simulink model "Table_airbus_v1"  (R2021b)
settings: Solver=VariableStepAuto  StartTime=0.0  StopTime=20  MaxStep=0.01  RelTol=0.01
undefined symbols (not defined in the file): X, Y, Z
libraries: sm_lib x907, fl_lib x69, nesl_utility x53, sdl_lib x10, ee_lib x7, slpidlib x6, simulink x5, simulink_extras x4
(part 16 of 18)

== system Table_airbus_v1/Modèle mécanique/Table/table_1_RIGID/x15060_M_01014_Ens_plateau_Default_1_RIGID/x15060_M_01003_Ens_structure_plateau_Default_1_RIGID ==
  ReferenceFrame : sm_lib/Frames and Transforms/Reference Frame
  Transform : sm_lib/Frames and Transforms/Rigid Transform  TranslationMethod=Cartesian  TranslationStandardOffset=0  TranslationLengthUnit=mm  TranslationStandardAxis=+Z  TranslationCartesianOffset=[860 265 20]  TranslationROffset=0  TranslationROffsetUnits=m  TranslationZOffset=0  TranslationZOffsetUnits=m  TranslationThetaOffset=0  TranslationThetaOffsetUnits=deg  RotationMethod=ArbitraryAxis  RotationAngleUnits=rad  RotationStandardAxis=+Z  RotationAngle=2.0943951023931953  RotationArbitraryAxis=[-0.57735026918962584 0.57735026918962584 0.57735026918962584]  FollAlignAxisA=+X  BaseAlignAxisA=+Y  FollAlignAxisB=+Y  BaseAlignAxisB=+Z  RotationSequenceAxes=FollowerAxes  RotationSequence=XYX  RotationSequenceAngles=[0 0 0]  RotationSequenceAnglesUnits=deg  RotationMatrix=[1 0 0; 0 1 0; 0 0 1]
  Transform1 : sm_lib/Frames and Transforms/Rigid Transform  TranslationMethod=Cartesian  TranslationStandardOffset=0  TranslationLengthUnit=mm  TranslationStandardAxis=+Z  TranslationCartesianOffset=[860 -375 0]  TranslationROffset=0  TranslationROffsetUnits=m  TranslationZOffset=0  TranslationZOffsetUnits=m  TranslationThetaOffset=0  TranslationThetaOffsetUnits=deg  RotationMethod=ArbitraryAxis  RotationAngleUnits=rad  RotationStandardAxis=+Z  RotationAngle=1.5707963267948968  RotationArbitraryAxis=[-5.5510999999999988e-17 5.5510999999999988e-17 1]  FollAlignAxisA=+X  BaseAlignAxisA=+Y  FollAlignAxisB=+Y  BaseAlignAxisB=+Z  RotationSequenceAxes=FollowerAxes  RotationSequence=XYX  RotationSequenceAngles=[0 0 0]  RotationSequenceAnglesUnits=deg  RotationMatrix=[1 0 0; 0 1 0; 0 0 1]
  Transform2 : sm_lib/Frames and Transforms/Rigid Transform  TranslationMethod=None  TranslationStandardOffset=0  TranslationLengthUnit=m  TranslationStandardAxis=+Z  TranslationCartesianOffset=[0 0 0]  TranslationROffset=0  TranslationROffsetUnits=m  TranslationZOffset=0  TranslationZOffsetUnits=m  TranslationThetaOffset=0  TranslationThetaOffsetUnits=deg  RotationMethod=None  RotationAngleUnits=deg  RotationStandardAxis=+Z  RotationAngle=0  RotationArbitraryAxis=[0 0 1]  FollAlignAxisA=+X  BaseAlignAxisA=+Y  FollAlignAxisB=+Y  BaseAlignAxisB=+Z  RotationSequenceAxes=FollowerAxes  RotationSequence=XYX  RotationSequenceAngles=[0 0 0]  RotationSequenceAnglesUnits=deg  RotationMatrix=[1 0 0; 0 1 0; 0 0 1]
  Transform3 : sm_lib/Frames and Transforms/Rigid Transform  TranslationMethod=Cartesian  TranslationStandardOffset=0  TranslationLengthUnit=mm  TranslationStandardAxis=+Z  TranslationCartesianOffset=[860 375 5.5217500000000003e-09]  TranslationROffset=0  TranslationROffsetUnits=m  TranslationZOffset=0  TranslationZOffsetUnits=m  TranslationThetaOffset=0  TranslationThetaOffsetUnits=deg  RotationMethod=ArbitraryAxis  RotationAngleUnits=rad  RotationStandardAxis=+Z  RotationAngle=3.1415926535897931  RotationArbitraryAxis=[0.70710678118654768 -0.70710678118654735 0]  FollAlignAxisA=+X  BaseAlignAxisA=+Y  FollAlignAxisB=+Y  BaseAlignAxisB=+Z  RotationSequenceAxes=FollowerAxes  RotationSequence=XYX  RotationSequenceAngles=[0 0 0]  RotationSequenceAnglesUnits=deg  RotationMatrix=[1 0 0; 0 1 0; 0 0 1]
  Transform4 : sm_lib/Frames and Transforms/Rigid Transform  TranslationMethod=None  TranslationStandardOffset=0  TranslationLengthUnit=m  TranslationStandardAxis=+Z  TranslationCartesianOffset=[0 0 0]  TranslationROffset=0  TranslationROffsetUnits=m  TranslationZOffset=0  TranslationZOffsetUnits=m  TranslationThetaOffset=0  TranslationThetaOffsetUnits=deg  RotationMethod=ArbitraryAxis  RotationAngleUnits=rad  RotationStandardAxis=+Z  RotationAngle=3.1415926535897931  RotationArbitraryAxis=[-6.3838000000000003e-16 1.3216950000000001e-15 -1]  FollAlignAxisA=+X  BaseAlignAxisA=+Y  FollAlignAxisB=+Y  BaseAlignAxisB=+Z  RotationSequenceAxes=FollowerAxes  RotationSequence=XYX  RotationSequenceAngles=[0 0 0]  RotationSequenceAnglesUnits=deg  RotationMatrix=[1 0 0; 0 1 0; 0 0 1]
  x15060_ITEM_Kit_Equerre_8_40x40_Zn_0_0_411_15_AA_DEFAULT_1_RIGI : Subsystem
  x15060_ITEM_Kit_Equerre_8_80x80_Zn_0_0_411_32_AA_DEFAULT_1_RIGI : Subsystem
  x15060_ITEM_Kit_Equerre_8_80x80_Zn_0_0_411_32_AA_DEFAULT_2_RIGI : Subsystem
  x15060_M_01021_Plateau_en_profil_alu_40x40_AA_DEFAULT_Brut_dusi : Subsystem
  F : PMIOPort  Side=Right
  connections:
  Transform4/LConn1 -- F/RConn1
  Transform4/RConn1 -- Transform3/LConn1 -- Transform2/LConn1 -- Transform1/LConn1 -- ReferenceFrame/RConn1 -- Transform/LConn1
  Transform3/RConn1 -- x15060_ITEM_Kit_Equerre_8_80x80_Zn_0_0_411_32_AA_DEFAULT_2_RIGI/LConn1
  Transform2/RConn1 -- x15060_M_01021_Plateau_en_profil_alu_40x40_AA_DEFAULT_Brut_dusi/LConn1
  Transform1/RConn1 -- x15060_ITEM_Kit_Equerre_8_80x80_Zn_0_0_411_32_AA_DEFAULT_1_RIGI/LConn1
  Transform/RConn1 -- x15060_ITEM_Kit_Equerre_8_40x40_Zn_0_0_411_15_AA_DEFAULT_1_RIGI/LConn1

== system Table_airbus_v1/Modèle mécanique/Table/table_1_RIGID/x15060_M_01014_Ens_plateau_Default_1_RIGID/x15060_M_01022_Plaque_sup_plateau_AA_DEFAULT_1_RIGID ==
  ReferenceFrame : sm_lib/Frames and Transforms/Reference Frame
  Solid : sm_lib/Body Elements/File Solid  ExtGeomFileName=15060-M-01022-Plaque sup plateau_AA - DEFAULT_Défaut_sldprt.STL  UnitType=Custom  ExtGeomFileUnits=mm  StepReaderType=HEX  ExportConvexHullGeometry=off  InertiaType=Custom  Mass=17.528600000000001  MassUnits=kg  CenterOfMass=[0 0 10.5]  CenterOfMassUnits=mm  MomentsOfInertia=[1002910 4728250 5729860]  MomentsOfInertiaUnits=kg*mm^2  ProductsOfInertia=[0 0 0]  ProductsOfInertiaUnits=kg*mm^2  BasedOnType=Density  Density=1000  DensityUnits=kg/(m^3)  DoExposeReferenceFrame=on  SerializedFrames=<Frames/>  GraphicType=FromGeometry  MarkerShape=Sphere  MarkerSize=10  MarkerSizeUnits=m  GraphicVisPropType=SimpleVisualProperties  GraphicDiffuseColor=[1 1 1]  GraphicSpecularColor=[0.5 0.5 0.5 1.0]  GraphicAmbientColor=[0.15 0.15 0.15 1.0]  GraphicEmissiveColor=[0.0 0.0 0.0 1.0]  GraphicShininess=75  GraphicOpacity=1
  F : PMIOPort  Side=Left
  connections:
  F/RConn1 -- ReferenceFrame/RConn1 -- Solid/RConn1

== system Table_airbus_v1/Modèle mécanique/Table/table_1_RIGID/x15060_M_01014_Ens_plateau_Default_1_RIGID/x15060_M_01024_Cale_reglet_AA_DEFAULT_1_RIGID ==
  ReferenceFrame : sm_lib/Frames and Transforms/Reference Frame
  Solid : sm_lib/Body Elements/File Solid  ExtGeomFileName=15060-M-01024-Cale reglet_AA - DEFAULT_Défaut_sldprt.STL  UnitType=Custom  ExtGeomFileUnits=mm  StepReaderType=HEX  ExportConvexHullGeometry=off  InertiaType=Custom  Mass=0.00835726  MassUnits=kg  CenterOfMass=[0 0 5]  CenterOfMassUnits=mm  MomentsOfInertia=[0.72748299999999999 0.68167800000000001 1.2698699999999998]  MomentsOfInertiaUnits=kg*mm^2  ProductsOfInertia=[0 0 0]  ProductsOfInertiaUnits=kg*mm^2  BasedOnType=Density  Density=1000  DensityUnits=kg/(m^3)  DoExposeReferenceFrame=on  SerializedFrames=<Frames/>  GraphicType=FromGeometry  MarkerShape=Sphere  MarkerSize=10  MarkerSizeUnits=m  GraphicVisPropType=SimpleVisualProperties  GraphicDiffuseColor=[0.792157 0.819608 0.933333]  GraphicSpecularColor=[0.5 0.5 0.5 1.0]  GraphicAmbientColor=[0.15 0.15 0.15 1.0]  GraphicEmissiveColor=[0.0 0.0 0.0 1.0]  GraphicShininess=75  GraphicOpacity=1
  F : PMIOPort  Side=Left
  connections:
  F/RConn1 -- ReferenceFrame/RConn1 -- Solid/RConn1

== system Table_airbus_v1/Modèle mécanique/Table/table_1_RIGID/x15060_M_01014_Ens_plateau_Default_1_RIGID/x15060_M_01032_Porte_pivot_AA_DEFAULT_1_RIGID ==
  ReferenceFrame : sm_lib/Frames and Transforms/Reference Frame
  Solid : sm_lib/Body Elements/File Solid  ExtGeomFileName=15060-M-01032-Porte pivot_AA - DEFAULT_Défaut_sldprt.STL  UnitType=Custom  ExtGeomFileUnits=mm  StepReaderType=HEX  ExportConvexHullGeometry=off  InertiaType=Custom  Mass=0.45541399999999999  MassUnits=kg  CenterOfMass=[-47.106400000000001 48.122499999999995 0.36210500000000001]  CenterOfMassUnits=mm  MomentsOfInertia=[388.97500000000002 432.13300000000004 691.03600000000006]  MomentsOfInertiaUnits=kg*mm^2  ProductsOfInertia=[-6.7267999999999999 6.8385800000000003 -294.24299999999999]  ProductsOfInertiaUnits=kg*mm^2  BasedOnType=Density  Density=1000  DensityUnits=kg/(m^3)  DoExposeReferenceFrame=on  SerializedFrames=<Frames/>  GraphicType=FromGeometry  MarkerShape=Sphere  MarkerSize=10  MarkerSizeUnits=m  GraphicVisPropType=SimpleVisualProperties  GraphicDiffuseColor=[0.898039 0.917647 0.929412]  GraphicSpecularColor=[0.5 0.5 0.5 1.0]  GraphicAmbientColor=[0.15 0.15 0.15 1.0]  GraphicEmissiveColor=[0.0 0.0 0.0 1.0]  GraphicShininess=75  GraphicOpacity=1
  F : PMIOPort  Side=Left
  connections:
  F/RConn1 -- ReferenceFrame/RConn1 -- Solid/RConn1

== system Table_airbus_v1/Modèle mécanique/Table/table_1_RIGID/x15060_M_01014_Ens_plateau_Default_1_RIGID/x15060_M_01034_Axe_pivot_AA_DEFAULT_1_RIGID ==
  ReferenceFrame : sm_lib/Frames and Transforms/Reference Frame
  Solid : sm_lib/Body Elements/File Solid  ExtGeomFileName=15060-M-01034-Axe pivot_AA - DEFAULT_Défaut_sldprt.STL  UnitType=Custom  ExtGeomFileUnits=mm  StepReaderType=HEX  ExportConvexHullGeometry=off  InertiaType=Custom  Mass=0.12033099999999999  MassUnits=kg  CenterOfMass=[0 0 0]  CenterOfMassUnits=mm  MomentsOfInertia=[3.38402 4651.21 4651.21]  MomentsOfInertiaUnits=kg*mm^2  ProductsOfInertia=[0 0 0]  ProductsOfInertiaUnits=kg*mm^2  BasedOnType=Density  Density=1000  DensityUnits=kg/(m^3)  DoExposeReferenceFrame=on  SerializedFrames=<Frames/>  GraphicType=FromGeometry  MarkerShape=Sphere  MarkerSize=10  MarkerSizeUnits=m  GraphicVisPropType=SimpleVisualProperties  GraphicDiffuseColor=[0.792157 0.819608 0.933333]  GraphicSpecularColor=[0.5 0.5 0.5 1.0]  GraphicAmbientColor=[0.15 0.15 0.15 1.0]  GraphicEmissiveColor=[0.0 0.0 0.0 1.0]  GraphicShininess=75  GraphicOpacity=1
  F : PMIOPort  Side=Left
  connections:
  F/RConn1 -- ReferenceFrame/RConn1 -- Solid/RConn1

== system Table_airbus_v1/Modèle mécanique/Table/table_1_RIGID/x15060_M_01014_Ens_plateau_Default_1_RIGID/x15060_M_01045_Articulation_2_AA_DEFAULT_1_RIGID ==
  ReferenceFrame : sm_lib/Frames and Transforms/Reference Frame
  Solid : sm_lib/Body Elements/File Solid  ExtGeomFileName=15060-M-01045-Articulation 2_AA - DEFAULT_Défaut_sldprt.STL  UnitType=Custom  ExtGeomFileUnits=mm  StepReaderType=HEX  ExportConvexHullGeometry=off  InertiaType=Custom  Mass=0.048731400000000001  MassUnits=kg  CenterOfMass=[-10.021800000000001 -22.492699999999999 -2.6463799999999999e-05]  CenterOfMassUnits=mm  MomentsOfInertia=[21.581199999999999 8.3179300000000005 22.579699999999999]  MomentsOfInertiaUnits=kg*mm^2  ProductsOfInertia=[2.3424100000000002e-05 1.00823e-07 4.5074899999999998]  ProductsOfInertiaUnits=kg*mm^2  BasedOnType=Density  Density=1000  DensityUnits=kg/(m^3)  DoExposeReferenceFrame=on  SerializedFrames=<Frames/>  GraphicType=FromGeometry  MarkerShape=Sphere  MarkerSize=10  MarkerSizeUnits=m  GraphicVisPropType=SimpleVisualProperties  GraphicDiffuseColor=[0.792157 0.819608 0.933333]  GraphicSpecularColor=[0.5 0.5 0.5 1.0]  GraphicAmbientColor=[0.15 0.15 0.15 1.0]  GraphicEmissiveColor=[0.0 0.0 0.0 1.0]  GraphicShininess=75  GraphicOpacity=1
  F : PMIOPort  Side=Left
  connections:
  F/RConn1 -- ReferenceFrame/RConn1 -- Solid/RConn1

== system Table_airbus_v1/Modèle mécanique/Table/table_1_RIGID/x15060_M_01014_Ens_plateau_Default_1_RIGID/x15060_M_01045_Articulation_2_AA_DEFAULT_2_RIGID ==
  ReferenceFrame : sm_lib/Frames and Transforms/Reference Frame
  Solid : sm_lib/Body Elements/File Solid  ExtGeomFileName=15060-M-01045-Articulation 2_AA - DEFAULT_Défaut_sldprt.STL  UnitType=Custom  ExtGeomFileUnits=mm  StepReaderType=HEX  ExportConvexHullGeometry=off  InertiaType=Custom  Mass=0.048731400000000001  MassUnits=kg  CenterOfMass=[-10.021800000000001 -22.492699999999999 -2.6463799999999999e-05]  CenterOfMassUnits=mm  MomentsOfInertia=[21.581199999999999 8.3179300000000005 22.579699999999999]  MomentsOfInertiaUnits=kg*mm^2  ProductsOfInertia=[2.3424100000000002e-05 1.00823e-07 4.5074899999999998]  ProductsOfInertiaUnits=kg*mm^2  BasedOnType=Density  Density=1000  DensityUnits=kg/(m^3)  DoExposeReferenceFrame=on  SerializedFrames=<Frames/>  GraphicType=FromGeometry  MarkerShape=Sphere  MarkerSize=10  MarkerSizeUnits=m  GraphicVisPropType=SimpleVisualProperties  GraphicDiffuseColor=[0.792157 0.819608 0.933333]  GraphicSpecularColor=[0.5 0.5 0.5 1.0]  GraphicAmbientColor=[0.15 0.15 0.15 1.0]  GraphicEmissiveColor=[0.0 0.0 0.0 1.0]  GraphicShininess=75  GraphicOpacity=1
  F : PMIOPort  Side=Left
  connections:
  F/RConn1 -- ReferenceFrame/RConn1 -- Solid/RConn1

== system Table_airbus_v1/Modèle mécanique/Table/table_1_RIGID/x15060_M_01014_Ens_plateau_Default_1_RIGID/x15060_M_01065_Porte_pivot_SYM_AA_DEFAULT_1_RIGID ==
  ReferenceFrame : sm_lib/Frames and Transforms/Reference Frame
  Solid : sm_lib/Body Elements/File Solid  ExtGeomFileName=15060-M-01065-Porte pivot - SYM_AA - DEFAULT_Défaut_sldprt.STL  UnitType=Custom  ExtGeomFileUnits=mm  StepReaderType=HEX  ExportConvexHullGeometry=off  InertiaType=Custom  Mass=0.45541399999999999  MassUnits=kg  CenterOfMass=[-47.106400000000001 48.122499999999995 -0.36212]  CenterOfMassUnits=mm  MomentsOfInertia=[388.97500000000002 432.13300000000004 691.03600000000006]  MomentsOfInertiaUnits=kg*mm^2  ProductsOfInertia=[6.72682 -6.8385300000000004 -294.24299999999999]  ProductsOfInertiaUnits=kg*mm^2  BasedOnType=Density  Density=1000  DensityUnits=kg/(m^3)  DoExposeReferenceFrame=on  SerializedFrames=<Frames/>  GraphicType=FromGeometry  MarkerShape=Sphere  MarkerSize=10  MarkerSizeUnits=m  GraphicVisPropType=SimpleVisualProperties  GraphicDiffuseColor=[0.898039 0.917647 0.929412]  GraphicSpecularColor=[0.5 0.5 0.5 1.0]  GraphicAmbientColor=[0.15 0.15 0.15 1.0]  GraphicEmissiveColor=[0.0 0.0 0.0 1.0]  GraphicShininess=75  GraphicOpacity=1
  F : PMIOPort  Side=Left
  connections:
  F/RConn1 -- ReferenceFrame/RConn1 -- Solid/RConn1

== system Table_airbus_v1/Modèle mécanique/Table/table_1_RIGID/x15060_M_01014_Ens_plateau_Default_1_RIGID/x15060_M_01072_Bloc_Rapporteur_angulaire_AA_DEFAULT_1_RIGID ==
  ReferenceFrame : sm_lib/Frames and Transforms/Reference Frame
  Solid : sm_lib/Body Elements/File Solid  ExtGeomFileName=15060-M-01072-Bloc Rapporteur angulaire_AA - DEFAULT_Défaut_sldprt.STL  UnitType=Custom  ExtGeomFileUnits=mm  StepReaderType=HEX  ExportConvexHullGeometry=off  InertiaType=Custom  Mass=0.0065508200000000006  MassUnits=kg  CenterOfMass=[2.0196800000000001 29.571099999999998 -36.991700000000002]  CenterOfMassUnits=mm  MomentsOfInertia=[2.33128 0.48933199999999993 1.85897]  MomentsOfInertiaUnits=kg*mm^2  ProductsOfInertia=[0.000850953 9.3975699999999989e-05 -0.0030936800000000001]  ProductsOfInertiaUnits=kg*mm^2  BasedOnType=Density  Density=1000  DensityUnits=kg/(m^3)  DoExposeReferenceFrame=on  SerializedFrames=<Frames/>  GraphicType=FromGeometry  MarkerShape=Sphere  MarkerSize=10  MarkerSizeUnits=m  GraphicVisPropType=SimpleVisualProperties  GraphicDiffuseColor=[0.792157 0.819608 0.933333]  GraphicSpecularColor=[0.5 0.5 0.5 1.0]  GraphicAmbientColor=[0.15 0.15 0.15 1.0]  GraphicEmissiveColor=[0.0 0.0 0.0 1.0]  GraphicShininess=75  GraphicOpacity=1
  F : PMIOPort  Side=Left
  connections:
  F/RConn1 -- ReferenceFrame/RConn1 -- Solid/RConn1

== system Table_airbus_v1/Modèle mécanique/Table/table_1_RIGID/x15060_M_01014_Ens_plateau_Default_1_RIGID/x15060_M_01082_Axe_pivot_avt_AA_DEFAULT_1_RIGID ==
  ReferenceFrame : sm_lib/Frames and Transforms/Reference Frame
  Solid : sm_lib/Body Elements/File Solid  ExtGeomFileName=15060-M-01082-Axe pivot avt_AA - DEFAULT_Défaut_sldprt.STL  UnitType=Custom  ExtGeomFileUnits=mm  StepReaderType=HEX  ExportConvexHullGeometry=off  InertiaType=Custom  Mass=0.0049980600000000003  MassUnits=kg  CenterOfMass=[-0.094775299999999993 0.0231576 0]  CenterOfMassUnits=mm  MomentsOfInertia=[0.08961269999999999 0.86225099999999999 0.86184300000000003]  MomentsOfInertiaUnits=kg*mm^2  ProductsOfInertia=[0 0 0.0021522199999999998]  ProductsOfInertiaUnits=kg*mm^2  BasedOnType=Density  Density=1000  DensityUnits=kg/(m^3)  DoExposeReferenceFrame=on  SerializedFrames=<Frames/>  GraphicType=FromGeometry  MarkerShape=Sphere  MarkerSize=10  MarkerSizeUnits=m  GraphicVisPropType=SimpleVisualProperties  GraphicDiffuseColor=[0.792157 0.819608 0.933333]  GraphicSpecularColor=[0.5 0.5 0.5 1.0]  GraphicAmbientColor=[0.15 0.15 0.15 1.0]  GraphicEmissiveColor=[0.0 0.0 0.0 1.0]  GraphicShininess=75  GraphicOpacity=1
  F : PMIOPort  Side=Left
  connections:
  F/RConn1 -- ReferenceFrame/RConn1 -- Solid/RConn1

== system Table_airbus_v1/Modèle mécanique/Table/table_1_RIGID/x15060_M_01014_Ens_plateau_Default_1_RIGID/x15060_M_01082_Axe_pivot_avt_AA_DEFAULT_2_RIGID ==
  ReferenceFrame : sm_lib/Frames and Transforms/Reference Frame
  Solid : sm_lib/Body Elements/File Solid  ExtGeomFileName=15060-M-01082-Axe pivot avt_AA - DEFAULT_Défaut_sldprt.STL  UnitType=Custom  ExtGeomFileUnits=mm  StepReaderType=HEX  ExportConvexHullGeometry=off  InertiaType=Custom  Mass=0.0049980600000000003  MassUnits=kg  CenterOfMass=[-0.094775299999999993 0.0231576 0]  CenterOfMassUnits=mm  MomentsOfInertia=[0.08961269999999999 0.86225099999999999 0.86184300000000003]  MomentsOfInertiaUnits=kg*mm^2  ProductsOfInertia=[0 0 0.0021522199999999998]  ProductsOfInertiaUnits=kg*mm^2  BasedOnType=Density  Density=1000  DensityUnits=kg/(m^3)  DoExposeReferenceFrame=on  SerializedFrames=<Frames/>  GraphicType=FromGeometry  MarkerShape=Sphere  MarkerSize=10  MarkerSizeUnits=m  GraphicVisPropType=SimpleVisualProperties  GraphicDiffuseColor=[0.792157 0.819608 0.933333]  GraphicSpecularColor=[0.5 0.5 0.5 1.0]  GraphicAmbientColor=[0.15 0.15 0.15 1.0]  GraphicEmissiveColor=[0.0 0.0 0.0 1.0]  GraphicShininess=75  GraphicOpacity=1
  F : PMIOPort  Side=Left
  connections:
  F/RConn1 -- ReferenceFrame/RConn1 -- Solid/RConn1

== system Table_airbus_v1/Modèle mécanique/Table/table_1_RIGID/x15060_M_01014_Ens_plateau_Default_1_RIGID/x15060_Rondelle_Rondelle_TresLarge_LL_5_1_RIGID ==
  ReferenceFrame : sm_lib/Frames and Transforms/Reference Frame
  Solid : sm_lib/Body Elements/File Solid  ExtGeomFileName=15060-Rondelle-_Rondelle TresLarge LL 5_Défaut_sldprt.STL  UnitType=Custom  ExtGeomFileUnits=mm  StepReaderType=HEX  ExportConvexHullGeometry=off  InertiaType=Custom  Mass=0.00029209700000000001  MassUnits=kg  CenterOfMass=[0 0.5 0]  CenterOfMassUnits=mm  MomentsOfInertia=[0.0078395899999999987 0.015630499999999999 0.0078395899999999987]  MomentsOfInertiaUnits=kg*mm^2  ProductsOfInertia=[0 0 0]  ProductsOfInertiaUnits=kg*mm^2  BasedOnType=Density  Density=1000  DensityUnits=kg/(m^3)  DoExposeReferenceFrame=on  SerializedFrames=<Frames/>  GraphicType=FromGeometry  MarkerShape=Sphere  MarkerSize=10  MarkerSizeUnits=m  GraphicVisPropType=SimpleVisualProperties  GraphicDiffuseColor=[0.792157 0.819608 0.933333]  GraphicSpecularColor=[0.5 0.5 0.5 1.0]  GraphicAmbientColor=[0.15 0.15 0.15 1.0]  GraphicEmissiveColor=[0.0 0.0 0.0 1.0]  GraphicShininess=75  GraphicOpacity=1
  F : PMIOPort  Side=Left
  connections:
  F/RConn1 -- ReferenceFrame/RConn1 -- Solid/RConn1

== system Table_airbus_v1/Modèle mécanique/Table/table_1_RIGID/x15060_M_01014_Ens_plateau_Default_1_RIGID/x15060_Vis_CHc_vis_CHc_M_5_X_8_1_RIGID ==
  ReferenceFrame : sm_lib/Frames and Transforms/Reference Frame
  Solid : sm_lib/Body Elements/File Solid  ExtGeomFileName="15060-Vis CHc-_vis CHc M 5 X   8_Défaut_sldprt.STL"  UnitType=Custom  ExtGeomFileUnits=mm  StepReaderType=HEX  ExportConvexHullGeometry=off  InertiaType=Custom  Mass=0.00039086999999999992  MassUnits=kg  CenterOfMass=[0 2.1901499999999999e-08 5.2160599999999997]  CenterOfMassUnits=mm  MomentsOfInertia=[0.0063825899999999996 0.0063838699999999998 0.00286112]  MomentsOfInertiaUnits=kg*mm^2  ProductsOfInertia=[0 0 -8.4326399999999992e-08]  ProductsOfInertiaUnits=kg*mm^2  BasedOnType=Density  Density=1000  DensityUnits=kg/(m^3)  DoExposeReferenceFrame=on  SerializedFrames=<Frames/>  GraphicType=FromGeometry  MarkerShape=Sphere  MarkerSize=10  MarkerSizeUnits=m  GraphicVisPropType=SimpleVisualProperties  GraphicDiffuseColor=[0.792157 0.819608 0.933333]  GraphicSpecularColor=[0.5 0.5 0.5 1.0]  GraphicAmbientColor=[0.15 0.15 0.15 1.0]  GraphicEmissiveColor=[0.0 0.0 0.0 1.0]  GraphicShininess=75  GraphicOpacity=1
  F : PMIOPort  Side=Left
  connections:
  F/RConn1 -- ReferenceFrame/RConn1 -- Solid/RConn1

== system Table_airbus_v1/Modèle mécanique/Table/table_1_RIGID/x15060_M_01018_Ch_ssis_haut_1_RIGID/x15060_Ecrou_22_Ecrou_Hm_M12_2_RIGID ==
  ReferenceFrame : sm_lib/Frames and Transforms/Reference Frame
  Solid : sm_lib/Body Elements/File Solid  ExtGeomFileName=15060-Ecrou-_22 - Ecrou Hm M12_Défaut_sldprt.STL  UnitType=Custom  ExtGeomFileUnits=mm  StepReaderType=HEX  ExportConvexHullGeometry=off  InertiaType=Custom  Mass=0.00136582  MassUnits=kg  CenterOfMass=[0 3 3.6598700000000002e-10]  CenterOfMassUnits=mm  MomentsOfInertia=[0.0470239 0.085997299999999999 0.0470239]  MomentsOfInertiaUnits=kg*mm^2  ProductsOfInertia=[0 0 0]  ProductsOfInertiaUnits=kg*mm^2  BasedOnType=Density  Density=1000  DensityUnits=kg/(m^3)  DoExposeReferenceFrame=on  SerializedFrames=<Frames/>  GraphicType=FromGeometry  MarkerShape=Sphere  MarkerSize=10  MarkerSizeUnits=m  GraphicVisPropType=SimpleVisualProperties  GraphicDiffuseColor=[0.792157 0.819608 0.933333]  GraphicSpecularColor=[0.5 0.5 0.5 1.0]  GraphicAmbientColor=[0.15 0.15 0.15 1.0]  GraphicEmissiveColor=[0.0 0.0 0.0 1.0]  GraphicShininess=75  GraphicOpacity=1
  F : PMIOPort  Side=Left
  connections:
  F/RConn1 -- ReferenceFrame/RConn1 -- Solid/RConn1

== system Table_airbus_v1/Modèle mécanique/Table/table_1_RIGID/x15060_M_01018_Ch_ssis_haut_1_RIGID/x15060_M_01015_Ens_verin_levage_Default_1_RIGID ==
  ReferenceFrame : sm_lib/Frames and Transforms/Reference Frame
  Transform : sm_lib/Frames and Transforms/Rigid Transform  TranslationMethod=Cartesian  TranslationStandardOffset=0  TranslationLengthUnit=mm  TranslationStandardAxis=+Z  TranslationCartesianOffset=[-517.07099999999991 35.420000000000002 16.307499999999997]  TranslationROffset=0  TranslationROffsetUnits=m  TranslationZOffset=0  TranslationZOffsetUnits=m  TranslationThetaOffset=0  TranslationThetaOffsetUnits=deg  RotationMethod=ArbitraryAxis  RotationAngleUnits=rad  RotationStandardAxis=+Z  RotationAngle=1.6424450276988594  RotationArbitraryAxis=[-0.25846666391264611 0.25846666391264667 -0.9308007129841136]  FollAlignAxisA=+X  BaseAlignAxisA=+Y  FollAlignAxisB=+Y  BaseAlignAxisB=+Z  RotationSequenceAxes=FollowerAxes  RotationSequence=XYX  RotationSequenceAngles=[0 0 0]  RotationSequenceAnglesUnits=deg  RotationMatrix=[1 0 0; 0 1 0; 0 0 1]
  F : PMIOPort  Side=Right
  connections:
  Transform/LConn1 -- F/RConn1
  ReferenceFrame/RConn1 -- Transform/RConn1

== system Table_airbus_v1/Modèle mécanique/Table/table_1_RIGID/x15060_M_01018_Ch_ssis_haut_1_RIGID/x15060_M_01016_Ens_verin_inclinaison_Default_1_RIGID ==
  ReferenceFrame : sm_lib/Frames and Transforms/Reference Frame
  Transform : sm_lib/Frames and Transforms/Rigid Transform  TranslationMethod=Cartesian  TranslationStandardOffset=0  TranslationLengthUnit=mm  TranslationStandardAxis=+Z  TranslationCartesianOffset=[-534.86299999999994 -149.5 81.105599999999995]  TranslationROffset=0  TranslationROffsetUnits=m  TranslationZOffset=0  TranslationZOffsetUnits=m  TranslationThetaOffset=0  TranslationThetaOffsetUnits=deg  RotationMethod=ArbitraryAxis  RotationAngleUnits=rad  RotationStandardAxis=+Z  RotationAngle=0.9229778637121423  RotationArbitraryAxis=[1.4239367345454361e-15 1 -3.9495448970531802e-16]  FollAlignAxisA=+X  BaseAlignAxisA=+Y  FollAlignAxisB=+Y  BaseAlignAxisB=+Z  RotationSequenceAxes=FollowerAxes  RotationSequence=XYX  RotationSequenceAngles=[0 0 0]  RotationSequenceAnglesUnits=deg  RotationMatrix=[1 0 0; 0 1 0; 0 0 1]
  F : PMIOPort  Side=Right
  connections:
  Transform/LConn1 -- F/RConn1
  ReferenceFrame/RConn1 -- Transform/RConn1

== system Table_airbus_v1/Modèle mécanique/Table/table_1_RIGID/x15060_M_01018_Ch_ssis_haut_1_RIGID/x15060_M_01025_Chape_sous_plateau_AA_DEFAULT_1_RIGID ==
  ReferenceFrame : sm_lib/Frames and Transforms/Reference Frame
  Solid : sm_lib/Body Elements/File Solid  ExtGeomFileName=15060-M-01025-Chape sous plateau_AA - DEFAULT_Défaut_sldprt.STL  UnitType=Custom  ExtGeomFileUnits=mm  StepReaderType=HEX  ExportConvexHullGeometry=off  InertiaType=Custom  Mass=10.1897  MassUnits=kg  CenterOfMass=[-52.1374 19.499599999999997 -14.3375]  CenterOfMassUnits=mm  MomentsOfInertia=[131905 115836 226896]  MomentsOfInertiaUnits=kg*mm^2  ProductsOfInertia=[-10849.700000000001 5459.5499999999993 -8876.1299999999992]  ProductsOfInertiaUnits=kg*mm^2  BasedOnType=Density  Density=1000  DensityUnits=kg/(m^3)  DoExposeReferenceFrame=on  SerializedFrames=<Frames/>  GraphicType=FromGeometry  MarkerShape=Sphere  MarkerSize=10  MarkerSizeUnits=m  GraphicVisPropType=SimpleVisualProperties  GraphicDiffuseColor=[0.776471 0.756863 0.737255]  GraphicSpecularColor=[0.5 0.5 0.5 1.0]  GraphicAmbientColor=[0.15 0.15 0.15 1.0]  GraphicEmissiveColor=[0.0 0.0 0.0 1.0]  GraphicShininess=75  GraphicOpacity=1
  F : PMIOPort  Side=Left
  connections:
  F/RConn1 -- ReferenceFrame/RConn1 -- Solid/RConn1

== system Table_airbus_v1/Modèle mécanique/Table/table_1_RIGID/x15060_M_01018_Ch_ssis_haut_1_RIGID/x15060_NLM_Vis_CHc_rectifi_e_a_paulement_16_L40_M12_07534_16x40 ==
  ReferenceFrame : sm_lib/Frames and Transforms/Reference Frame
  Solid : sm_lib/Body Elements/File Solid  ExtGeomFileName=15060-NLM-Vis CHc rectifieapaulement I16 - DEFAULT_Défaut_sldprt.STL  UnitType=Custom  ExtGeomFileUnits=mm  StepReaderType=HEX  ExportConvexHullGeometry=off  InertiaType=Custom  Mass=0.113359  MassUnits=kg  CenterOfMass=[16.023200000000003 0 0]  CenterOfMassUnits=mm  MomentsOfInertia=[4.9999099999999999 45.857199999999999 45.857199999999999]  MomentsOfInertiaUnits=kg*mm^2  ProductsOfInertia=[0 0 0]  ProductsOfInertiaUnits=kg*mm^2  BasedOnType=Density  Density=1000  DensityUnits=kg/(m^3)  DoExposeReferenceFrame=on  SerializedFrames=<Frames/>  GraphicType=FromGeometry  MarkerShape=Sphere  MarkerSize=10  MarkerSizeUnits=m  GraphicVisPropType=SimpleVisualProperties  GraphicDiffuseColor=[0.776471 0.756863 0.737255]  GraphicSpecularColor=[0.5 0.5 0.5 1.0]  GraphicAmbientColor=[0.15 0.15 0.15 1.0]  GraphicEmissiveColor=[0.0 0.0 0.0 1.0]  GraphicShininess=75  GraphicOpacity=1
  F : PMIOPort  Side=Left
  connections:
  F/RConn1 -- Solid/RConn1 -- ReferenceFrame/RConn1

== system Table_airbus_v1/Modèle mécanique/Table/table_1_RIGID/x15060_M_01018_Ch_ssis_haut_1_RIGID/x15060_Rondelle_Rondelle_TresLarge_LL_6_1_RIGID ==
  ReferenceFrame : sm_lib/Frames and Transforms/Reference Frame
  Solid : sm_lib/Body Elements/File Solid  ExtGeomFileName=15060-Rondelle-_Rondelle TresLarge LL 6_Défaut_sldprt.STL  UnitType=Custom  ExtGeomFileUnits=mm  StepReaderType=HEX  ExportConvexHullGeometry=off  InertiaType=Custom  Mass=0.00050426300000000002  MassUnits=kg  CenterOfMass=[0 0.60000000000000009 0]  CenterOfMassUnits=mm  MomentsOfInertia=[0.019504899999999999 0.038888800000000001 0.019504899999999999]  MomentsOfInertiaUnits=kg*mm^2  ProductsOfInertia=[0 0 0]  ProductsOfInertiaUnits=kg*mm^2  BasedOnType=Density  Density=1000  DensityUnits=kg/(m^3)  DoExposeReferenceFrame=on  SerializedFrames=<Frames/>  GraphicType=FromGeometry  MarkerShape=Sphere  MarkerSize=10  MarkerSizeUnits=m  GraphicVisPropType=SimpleVisualProperties  GraphicDiffuseColor=[0.792157 0.819608 0.933333]  GraphicSpecularColor=[0.5 0.5 0.5 1.0]  GraphicAmbientColor=[0.15 0.15 0.15 1.0]  GraphicEmissiveColor=[0.0 0.0 0.0 1.0]  GraphicShininess=75  GraphicOpacity=1
  F : PMIOPort  Side=Left
  connections:
  F/RConn1 -- ReferenceFrame/RConn1 -- Solid/RConn1

== system Table_airbus_v1/Modèle mécanique/Table/table_1_RIGID/x15060_M_01018_Ch_ssis_haut_1_RIGID/x15060_Vis_CHc_vis_CHc_M_6_X_10_1_RIGID ==
  ReferenceFrame : sm_lib/Frames and Transforms/Reference Frame
  Solid : sm_lib/Body Elements/File Solid  ExtGeomFileName="15060-Vis CHc-_vis CHc M 6 X  10_Défaut_sldprt.STL"  UnitType=Custom  ExtGeomFileUnits=mm  StepReaderType=HEX  ExportConvexHullGeometry=off  InertiaType=Custom  Mass=0.00066133499999999998  MassUnits=kg  CenterOfMass=[0 2.5945499999999999e-08 6.5531500000000005]  CenterOfMassUnits=mm  MomentsOfInertia=[0.016208500000000001 0.016211699999999999 0.0066540999999999996]  MomentsOfInertiaUnits=kg*mm^2  ProductsOfInertia=[0 0 -3.1329799999999998e-07]  ProductsOfInertiaUnits=kg*mm^2  BasedOnType=Density  Density=1000  DensityUnits=kg/(m^3)  DoExposeReferenceFrame=on  SerializedFrames=<Frames/>  GraphicType=FromGeometry  MarkerShape=Sphere  MarkerSize=10  MarkerSizeUnits=m  GraphicVisPropType=SimpleVisualProperties  GraphicDiffuseColor=[0.792157 0.819608 0.933333]  GraphicSpecularColor=[0.5 0.5 0.5 1.0]  GraphicAmbientColor=[0.15 0.15 0.15 1.0]  GraphicEmissiveColor=[0.0 0.0 0.0 1.0]  GraphicShininess=75  GraphicOpacity=1
  F : PMIOPort  Side=Left
  connections:
  F/RConn1 -- ReferenceFrame/RConn1 -- Solid/RConn1

== system Table_airbus_v1/Modèle mécanique/Table/table_1_RIGID/x15060_M_01002_Ens_cadre_Default_1_RIGID/x15060_M_01004_Ens_barre_de_cadre_1_Default_1_RIGID/x15060_M_01041_Plaquette_sur_glissiere_AA_DEFAULT_1_RIGID ==
  ReferenceFrame : sm_lib/Frames and Transforms/Reference Frame
  Solid : sm_lib/Body Elements/File Solid  ExtGeomFileName=15060-M-01041-Plaquette sur glissiere_AA - DEFAULT_Défaut_sldprt.STL  UnitType=Custom  ExtGeomFileUnits=mm  StepReaderType=HEX  ExportConvexHullGeometry=off  InertiaType=Custom  Mass=0.066996899999999998  MassUnits=kg  CenterOfMass=[-1.5298499999999999 -0.085960300000000003 4.9779900000000001]  CenterOfMassUnits=mm  MomentsOfInertia=[7.6590700000000007 34.768699999999995 41.3262]  MomentsOfInertiaUnits=kg*mm^2  ProductsOfInertia=[-0.0011722600000000001 -0.039111800000000002 -0.014471899999999999]  ProductsOfInertiaUnits=kg*mm^2  BasedOnType=Density  Density=1000  DensityUnits=kg/(m^3)  DoExposeReferenceFrame=on  SerializedFrames=<Frames/>  GraphicType=FromGeometry  MarkerShape=Sphere  MarkerSize=10  MarkerSizeUnits=m  GraphicVisPropType=SimpleVisualProperties  GraphicDiffuseColor=[0.898039 0.917647 0.929412]  GraphicSpecularColor=[0.5 0.5 0.5 1.0]  GraphicAmbientColor=[0.15 0.15 0.15 1.0]  GraphicEmissiveColor=[0.0 0.0 0.0 1.0]  GraphicShininess=75  GraphicOpacity=1
  F : PMIOPort  Side=Left
  connections:
  F/RConn1 -- ReferenceFrame/RConn1 -- Solid/RConn1

== system Table_airbus_v1/Modèle mécanique/Table/table_1_RIGID/x15060_M_01002_Ens_cadre_Default_1_RIGID/x15060_M_01004_Ens_barre_de_cadre_1_Default_1_RIGID/x15060_M_01042_Barre_transversale_AA_DEFAULT_1_RIGID ==
  ReferenceFrame : sm_lib/Frames and Transforms/Reference Frame
  Solid : sm_lib/Body Elements/File Solid  ExtGeomFileName=15060-M-01042-Barre transversale_AA - DEFAULT_Défaut_sldprt.STL  UnitType=Custom  ExtGeomFileUnits=mm  StepReaderType=HEX  ExportConvexHullGeometry=off  InertiaType=Custom  Mass=0.60250400000000004  MassUnits=kg  CenterOfMass=[0 0 -1.04198e-12]  CenterOfMassUnits=mm  MomentsOfInertia=[20808.599999999999 20753.200000000001 65.337600000000009]  MomentsOfInertiaUnits=kg*mm^2  ProductsOfInertia=[0 0 0]  ProductsOfInertiaUnits=kg*mm^2  BasedOnType=Density  Density=1000  DensityUnits=kg/(m^3)  DoExposeReferenceFrame=on  SerializedFrames=<Frames/>  GraphicType=FromGeometry  MarkerShape=Sphere  MarkerSize=10  MarkerSizeUnits=m  GraphicVisPropType=SimpleVisualProperties  GraphicDiffuseColor=[0.898039 0.917647 0.929412]  GraphicSpecularColor=[0.5 0.5 0.5 1.0]  GraphicAmbientColor=[0.15 0.15 0.15 1.0]  GraphicEmissiveColor=[0.0 0.0 0.0 1.0]  GraphicShininess=75  GraphicOpacity=1
  F : PMIOPort  Side=Left
  connections:
  F/RConn1 -- ReferenceFrame/RConn1 -- Solid/RConn1

== system Table_airbus_v1/Modèle mécanique/Table/table_1_RIGID/x15060_M_01002_Ens_cadre_Default_1_RIGID/x15060_M_01004_Ens_barre_de_cadre_1_Default_1_RIGID/x15060_M_01043_Bride_de_barre_AA_DEFAULT_1_RIGID ==
  ReferenceFrame : sm_lib/Frames and Transforms/Reference Frame
  Solid : sm_lib/Body Elements/File Solid  ExtGeomFileName=15060-M-01043-Bride de barre_AA - DEFAULT_Défaut_sldprt.STL  UnitType=Custom  ExtGeomFileUnits=mm  StepReaderType=HEX  ExportConvexHullGeometry=off  InertiaType=Custom  Mass=0.0646534  MassUnits=kg  CenterOfMass=[0 -0.40050599999999997 5.0587200000000001]  CenterOfMassUnits=mm  MomentsOfInertia=[5.7510300000000001 34.636699999999998 39.315600000000003]  MomentsOfInertiaUnits=kg*mm^2  ProductsOfInertia=[0.038467100000000004 0 0]  ProductsOfInertiaUnits=kg*mm^2  BasedOnType=Density  Density=1000  DensityUnits=kg/(m^3)  DoExposeReferenceFrame=on  SerializedFrames=<Frames/>  GraphicType=FromGeometry  MarkerShape=Sphere  MarkerSize=10  MarkerSizeUnits=m  GraphicVisPropType=SimpleVisualProperties  GraphicDiffuseColor=[0.898039 0.917647 0.929412]  GraphicSpecularColor=[0.5 0.5 0.5 1.0]  GraphicAmbientColor=[0.15 0.15 0.15 1.0]  GraphicEmissiveColor=[0.0 0.0 0.0 1.0]  GraphicShininess=75  GraphicOpacity=1
  F : PMIOPort  Side=Left
  connections:
  F/RConn1 -- ReferenceFrame/RConn1 -- Solid/RConn1

== system Table_airbus_v1/Modèle mécanique/Table/table_1_RIGID/x15060_M_01002_Ens_cadre_Default_1_RIGID/x15060_M_01004_Ens_barre_de_cadre_1_Default_1_RIGID/x15060_M_01043_Bride_de_barre_AA_DEFAULT_2_RIGID ==
  ReferenceFrame : sm_lib/Frames and Transforms/Reference Frame
  Solid : sm_lib/Body Elements/File Solid  ExtGeomFileName=15060-M-01043-Bride de barre_AA - DEFAULT_Défaut_sldprt.STL  UnitType=Custom  ExtGeomFileUnits=mm  StepReaderType=HEX  ExportConvexHullGeometry=off  InertiaType=Custom  Mass=0.0646534  MassUnits=kg  CenterOfMass=[0 -0.40050599999999997 5.0587200000000001]  CenterOfMassUnits=mm  MomentsOfInertia=[5.7510300000000001 34.636699999999998 39.315600000000003]  MomentsOfInertiaUnits=kg*mm^2  ProductsOfInertia=[0.038467100000000004 0 0]  ProductsOfInertiaUnits=kg*mm^2  BasedOnType=Density  Density=1000  DensityUnits=kg/(m^3)  DoExposeReferenceFrame=on  SerializedFrames=<Frames/>  GraphicType=FromGeometry  MarkerShape=Sphere  MarkerSize=10  MarkerSizeUnits=m  GraphicVisPropType=SimpleVisualProperties  GraphicDiffuseColor=[0.898039 0.917647 0.929412]  GraphicSpecularColor=[0.5 0.5 0.5 1.0]  GraphicAmbientColor=[0.15 0.15 0.15 1.0]  GraphicEmissiveColor=[0.0 0.0 0.0 1.0]  GraphicShininess=75  GraphicOpacity=1
  F : PMIOPort  Side=Left
  connections:
  F/RConn1 -- ReferenceFrame/RConn1 -- Solid/RConn1

== system Table_airbus_v1/Modèle mécanique/Table/table_1_RIGID/x15060_M_01002_Ens_cadre_Default_1_RIGID/x15060_M_01004_Ens_barre_de_cadre_1_Default_1_RIGID/x15060_M_01051_Plaquette_sur_glissiere_SYM_AA_DEFAULT_1_RIGID ==
  ReferenceFrame : sm_lib/Frames and Transforms/Reference Frame
  Solid : sm_lib/Body Elements/File Solid  ExtGeomFileName=15060-M-01051-Plaquette sur glissiere - SYM_AA - DEFAULT_Défaut_sldprt.STL  UnitType=Custom  ExtGeomFileUnits=mm  StepReaderType=HEX  ExportConvexHullGeometry=off  InertiaType=Custom  Mass=0.066997100000000004  MassUnits=kg  CenterOfMass=[-1.5299699999999998 -0.085981099999999991 -4.9779900000000001]  CenterOfMassUnits=mm  MomentsOfInertia=[7.6590799999999994 34.768699999999995 41.326299999999996]  MomentsOfInertiaUnits=kg*mm^2  ProductsOfInertia=[0.0011704100000000002 0.039114500000000003 -0.014373]  ProductsOfInertiaUnits=kg*mm^2  BasedOnType=Density  Density=1000  DensityUnits=kg/(m^3)  DoExposeReferenceFrame=on  SerializedFrames=<Frames/>  GraphicType=FromGeometry  MarkerShape=Sphere  MarkerSize=10  MarkerSizeUnits=m  GraphicVisPropType=SimpleVisualProperties  GraphicDiffuseColor=[0.898039 0.917647 0.929412]  GraphicSpecularColor=[0.5 0.5 0.5 1.0]  GraphicAmbientColor=[0.15 0.15 0.15 1.0]  GraphicEmissiveColor=[0.0 0.0 0.0 1.0]  GraphicShininess=75  GraphicOpacity=1
  F : PMIOPort  Side=Left
  connections:
  F/RConn1 -- ReferenceFrame/RConn1 -- Solid/RConn1

== system Table_airbus_v1/Modèle mécanique/Table/table_1_RIGID/x15060_M_01002_Ens_cadre_Default_1_RIGID/x15060_M_01004_Ens_barre_de_cadre_1_Default_1_RIGID/x15060_NLM_Goupille_cyl_3_Lgr_16_03320_03x16_AA_DEFAULT_1_RIGID ==
  ReferenceFrame : sm_lib/Frames and Transforms/Reference Frame
  Solid : sm_lib/Body Elements/File Solid  ExtGeomFileName=15060-NLM-Goupille cyl I3 Lgr 16 - 03320-03x16_AA - DEFAULT_Défaut_sldprt.STL  UnitType=Custom  ExtGeomFileUnits=mm  StepReaderType=HEX  ExportConvexHullGeometry=off  InertiaType=Custom  Mass=0.000113097  MassUnits=kg  CenterOfMass=[8 0 0]  CenterOfMassUnits=mm  MomentsOfInertia=[0.00012723500000000001 0.0024763599999999999 0.0024763599999999999]  MomentsOfInertiaUnits=kg*mm^2  ProductsOfInertia=[0 0 0]  ProductsOfInertiaUnits=kg*mm^2  BasedOnType=Density  Density=1000  DensityUnits=kg/(m^3)  DoExposeReferenceFrame=on  SerializedFrames=<Frames/>  GraphicType=FromGeometry  MarkerShape=Sphere  MarkerSize=10  MarkerSizeUnits=m  GraphicVisPropType=SimpleVisualProperties  GraphicDiffuseColor=[0.792157 0.819608 0.933333]  GraphicSpecularColor=[0.5 0.5 0.5 1.0]  GraphicAmbientColor=[0.15 0.15 0.15 1.0]  GraphicEmissiveColor=[0.0 0.0 0.0 1.0]  GraphicShininess=75  GraphicOpacity=1
  F : PMIOPort  Side=Left
  connections:
  F/RConn1 -- Solid/RConn1 -- ReferenceFrame/RConn1

== system Table_airbus_v1/Modèle mécanique/Table/table_1_RIGID/x15060_M_01002_Ens_cadre_Default_1_RIGID/x15060_M_01004_Ens_barre_de_cadre_1_Default_1_RIGID/x15060_NLM_Goupille_cyl_3_Lgr_16_03320_03x16_AA_DEFAULT_2_RIGID ==
  ReferenceFrame : sm_lib/Frames and Transforms/Reference Frame
  Solid : sm_lib/Body Elements/File Solid  ExtGeomFileName=15060-NLM-Goupille cyl I3 Lgr 16 - 03320-03x16_AA - DEFAULT_Défaut_sldprt.STL  UnitType=Custom  ExtGeomFileUnits=mm  StepReaderType=HEX  ExportConvexHullGeometry=off  InertiaType=Custom  Mass=0.000113097  MassUnits=kg  CenterOfMass=[8 0 0]  CenterOfMassUnits=mm  MomentsOfInertia=[0.00012723500000000001 0.0024763599999999999 0.0024763599999999999]  MomentsOfInertiaUnits=kg*mm^2  ProductsOfInertia=[0 0 0]  ProductsOfInertiaUnits=kg*mm^2  BasedOnType=Density  Density=1000  DensityUnits=kg/(m^3)  DoExposeReferenceFrame=on  SerializedFrames=<Frames/>  GraphicType=FromGeometry  MarkerShape=Sphere  MarkerSize=10  MarkerSizeUnits=m  GraphicVisPropType=SimpleVisualProperties  GraphicDiffuseColor=[0.792157 0.819608 0.933333]  GraphicSpecularColor=[0.5 0.5 0.5 1.0]  GraphicAmbientColor=[0.15 0.15 0.15 1.0]  GraphicEmissiveColor=[0.0 0.0 0.0 1.0]  GraphicShininess=75  GraphicOpacity=1
  F : PMIOPort  Side=Left
  connections:
  F/RConn1 -- Solid/RConn1 -- ReferenceFrame/RConn1

== system Table_airbus_v1/Modèle mécanique/Table/table_1_RIGID/x15060_M_01002_Ens_cadre_Default_1_RIGID/x15060_M_01004_Ens_barre_de_cadre_1_Default_1_RIGID/x15060_NLM_Poign_e_Miniwing_M6_06652_006_X_15_1_RIGID ==
  ReferenceFrame : sm_lib/Frames and Transforms/Reference Frame
  Solid : sm_lib/Body Elements/File Solid  ExtGeomFileName=15060-NLM-Poignee Miniwing M6 - 06652-006 X 15_Défaut_sldprt.STL  UnitType=Custom  ExtGeomFileUnits=mm  StepReaderType=HEX  ExportConvexHullGeometry=off  InertiaType=Custom  Mass=0.0031415499999999999  MassUnits=kg  CenterOfMass=[0 5.4933500000000004 0]  CenterOfMassUnits=mm  MomentsOfInertia=[0.151592 0.116684 0.22078500000000001]  MomentsOfInertiaUnits=kg*mm^2  ProductsOfInertia=[0 0.0064548499999999998 0]  ProductsOfInertiaUnits=kg*mm^2  BasedOnType=Density  Density=1000  DensityUnits=kg/(m^3)  DoExposeReferenceFrame=on  SerializedFrames=<Frames/>  GraphicType=FromGeometry  MarkerShape=Sphere  MarkerSize=10  MarkerSizeUnits=m  GraphicVisPropType=SimpleVisualProperties  GraphicDiffuseColor=[0.792157 0.819608 0.933333]  GraphicSpecularColor=[0.5 0.5 0.5 1.0]  GraphicAmbientColor=[0.15 0.15 0.15 1.0]  GraphicEmissiveColor=[0.0 0.0 0.0 1.0]  GraphicShininess=75  GraphicOpacity=1
  F : PMIOPort  Side=Left
  connections:
  F/RConn1 -- Solid/RConn1 -- ReferenceFrame/RConn1

== system Table_airbus_v1/Modèle mécanique/Table/table_1_RIGID/x15060_M_01002_Ens_cadre_Default_1_RIGID/x15060_M_01004_Ens_barre_de_cadre_1_Default_1_RIGID/x15060_NLM_Poign_e_Miniwing_M6_06652_006_X_15_2_RIGID ==
  ReferenceFrame : sm_lib/Frames and Transforms/Reference Frame
  Solid : sm_lib/Body Elements/File Solid  ExtGeomFileName=15060-NLM-Poignee Miniwing M6 - 06652-006 X 15_Défaut_sldprt.STL  UnitType=Custom  ExtGeomFileUnits=mm  StepReaderType=HEX  ExportConvexHullGeometry=off  InertiaType=Custom  Mass=0.0031415499999999999  MassUnits=kg  CenterOfMass=[0 5.4933500000000004 0]  CenterOfMassUnits=mm  MomentsOfInertia=[0.151592 0.116684 0.22078500000000001]  MomentsOfInertiaUnits=kg*mm^2  ProductsOfInertia=[0 0.0064548499999999998 0]  ProductsOfInertiaUnits=kg*mm^2  BasedOnType=Density  Density=1000  DensityUnits=kg/(m^3)  DoExposeReferenceFrame=on  SerializedFrames=<Frames/>  GraphicType=FromGeometry  MarkerShape=Sphere  MarkerSize=10  MarkerSizeUnits=m  GraphicVisPropType=SimpleVisualProperties  GraphicDiffuseColor=[0.792157 0.819608 0.933333]  GraphicSpecularColor=[0.5 0.5 0.5 1.0]  GraphicAmbientColor=[0.15 0.15 0.15 1.0]  GraphicEmissiveColor=[0.0 0.0 0.0 1.0]  GraphicShininess=75  GraphicOpacity=1
  F : PMIOPort  Side=Left
  connections:
  F/RConn1 -- Solid/RConn1 -- ReferenceFrame/RConn1

== system Table_airbus_v1/Modèle mécanique/Table/table_1_RIGID/x15060_M_01002_Ens_cadre_Default_1_RIGID/x15060_M_01004_Ens_barre_de_cadre_1_Default_1_RIGID/x15060_Rondelle_Rondelle_Etroite_Z_4_1_RIGID ==
  ReferenceFrame : sm_lib/Frames and Transforms/Reference Frame
  Solid : sm_lib/Body Elements/File Solid  ExtGeomFileName=15060-Rondelle-_Rondelle Etroite Z 4_Défaut_sldprt.STL  UnitType=Custom  ExtGeomFileUnits=mm  StepReaderType=HEX  ExportConvexHullGeometry=off  InertiaType=Custom  Mass=3.9276200000000002e-05  MassUnits=kg  CenterOfMass=[0 0.40000000000000002 0]  CenterOfMassUnits=mm  MomentsOfInertia=[0.000246319 0.00048844899999999996 0.000246319]  MomentsOfInertiaUnits=kg*mm^2  ProductsOfInertia=[0 0 0]  ProductsOfInertiaUnits=kg*mm^2  BasedOnType=Density  Density=1000  DensityUnits=kg/(m^3)  DoExposeReferenceFrame=on  SerializedFrames=<Frames/>  GraphicType=FromGeometry  MarkerShape=Sphere  MarkerSize=10  MarkerSizeUnits=m  GraphicVisPropType=SimpleVisualProperties  GraphicDiffuseColor=[0.792157 0.819608 0.933333]  GraphicSpecularColor=[0.5 0.5 0.5 1.0]  GraphicAmbientColor=[0.15 0.15 0.15 1.0]  GraphicEmissiveColor=[0.0 0.0 0.0 1.0]  GraphicShininess=75  GraphicOpacity=1
  F : PMIOPort  Side=Left
  connections:
  F/RConn1 -- ReferenceFrame/RConn1 -- Solid/RConn1

== system Table_airbus_v1/Modèle mécanique/Table/table_1_RIGID/x15060_M_01002_Ens_cadre_Default_1_RIGID/x15060_M_01004_Ens_barre_de_cadre_1_Default_1_RIGID/x15060_Rondelle_Rondelle_Etroite_Z_4_2_RIGID ==
  ReferenceFrame : sm_lib/Frames and Transforms/Reference Frame
  Solid : sm_lib/Body Elements/File Solid  ExtGeomFileName=15060-Rondelle-_Rondelle Etroite Z 4_Défaut_sldprt.STL  UnitType=Custom  ExtGeomFileUnits=mm  StepReaderType=HEX  ExportConvexHullGeometry=off  InertiaType=Custom  Mass=3.9276200000000002e-05  MassUnits=kg  CenterOfMass=[0 0.40000000000000002 0]  CenterOfMassUnits=mm  MomentsOfInertia=[0.000246319 0.00048844899999999996 0.000246319]  MomentsOfInertiaUnits=kg*mm^2  ProductsOfInertia=[0 0 0]  ProductsOfInertiaUnits=kg*mm^2  BasedOnType=Density  Density=1000  DensityUnits=kg/(m^3)  DoExposeReferenceFrame=on  SerializedFrames=<Frames/>  GraphicType=FromGeometry  MarkerShape=Sphere  MarkerSize=10  MarkerSizeUnits=m  GraphicVisPropType=SimpleVisualProperties  GraphicDiffuseColor=[0.792157 0.819608 0.933333]  GraphicSpecularColor=[0.5 0.5 0.5 1.0]  GraphicAmbientColor=[0.15 0.15 0.15 1.0]  GraphicEmissiveColor=[0.0 0.0 0.0 1.0]  GraphicShininess=75  GraphicOpacity=1
  F : PMIOPort  Side=Left
  connections:
  F/RConn1 -- ReferenceFrame/RConn1 -- Solid/RConn1

== system Table_airbus_v1/Modèle mécanique/Table/table_1_RIGID/x15060_M_01002_Ens_cadre_Default_1_RIGID/x15060_M_01004_Ens_barre_de_cadre_1_Default_1_RIGID/x15060_Rondelle_Rondelle_Etroite_Z_4_3_RIGID ==
  ReferenceFrame : sm_lib/Frames and Transforms/Reference Frame
  Solid : sm_lib/Body Elements/File Solid  ExtGeomFileName=15060-Rondelle-_Rondelle Etroite Z 4_Défaut_sldprt.STL  UnitType=Custom  ExtGeomFileUnits=mm  StepReaderType=HEX  ExportConvexHullGeometry=off  InertiaType=Custom  Mass=3.9276200000000002e-05  MassUnits=kg  CenterOfMass=[0 0.40000000000000002 0]  CenterOfMassUnits=mm  MomentsOfInertia=[0.000246319 0.00048844899999999996 0.000246319]  MomentsOfInertiaUnits=kg*mm^2  ProductsOfInertia=[0 0 0]  ProductsOfInertiaUnits=kg*mm^2  BasedOnType=Density  Density=1000  DensityUnits=kg/(m^3)  DoExposeReferenceFrame=on  SerializedFrames=<Frames/>  GraphicType=FromGeometry  MarkerShape=Sphere  MarkerSize=10  MarkerSizeUnits=m  GraphicVisPropType=SimpleVisualProperties  GraphicDiffuseColor=[0.792157 0.819608 0.933333]  GraphicSpecularColor=[0.5 0.5 0.5 1.0]  GraphicAmbientColor=[0.15 0.15 0.15 1.0]  GraphicEmissiveColor=[0.0 0.0 0.0 1.0]  GraphicShininess=75  GraphicOpacity=1
  F : PMIOPort  Side=Left
  connections:
  F/RConn1 -- ReferenceFrame/RConn1 -- Solid/RConn1

== system Table_airbus_v1/Modèle mécanique/Table/table_1_RIGID/x15060_M_01002_Ens_cadre_Default_1_RIGID/x15060_M_01004_Ens_barre_de_cadre_1_Default_1_RIGID/x15060_Vis_CHc_vis_CHc_M_4_X_12_1_RIGID ==
  ReferenceFrame : sm_lib/Frames and Transforms/Reference Frame
  Solid : sm_lib/Body Elements/File Solid  ExtGeomFileName="15060-Vis CHc-_vis CHc M 4 X  12_Défaut_sldprt.STL"  UnitType=Custom  ExtGeomFileUnits=mm  StepReaderType=HEX  ExportConvexHullGeometry=off  InertiaType=Custom  Mass=0.00028164600000000003  MassUnits=kg  CenterOfMass=[0 1.2813e-08 6.3179499999999997]  CenterOfMassUnits=mm  MomentsOfInertia=[0.0068365400000000003 0.0068372900000000002 0.00118534]  MomentsOfInertiaUnits=kg*mm^2  ProductsOfInertia=[0 0 -4.9500699999999998e-08]  ProductsOfInertiaUnits=kg*mm^2  BasedOnType=Density  Density=1000  DensityUnits=kg/(m^3)  DoExposeReferenceFrame=on  SerializedFrames=<Frames/>  GraphicType=FromGeometry  MarkerShape=Sphere  MarkerSize=10  MarkerSizeUnits=m  GraphicVisPropType=SimpleVisualProperties  GraphicDiffuseColor=[0.792157 0.819608 0.933333]  GraphicSpecularColor=[0.5 0.5 0.5 1.0]  GraphicAmbientColor=[0.15 0.15 0.15 1.0]  GraphicEmissiveColor=[0.0 0.0 0.0 1.0]  GraphicShininess=75  GraphicOpacity=1
  F : PMIOPort  Side=Left
  connections:
  F/RConn1 -- ReferenceFrame/RConn1 -- Solid/RConn1

== system Table_airbus_v1/Modèle mécanique/Table/table_1_RIGID/x15060_M_01002_Ens_cadre_Default_1_RIGID/x15060_M_01004_Ens_barre_de_cadre_1_Default_1_RIGID/x15060_Vis_CHc_vis_CHc_M_4_X_16_1_RIGID ==
  ReferenceFrame : sm_lib/Frames and Transforms/Reference Frame
  Solid : sm_lib/Body Elements/File Solid  ExtGeomFileName="15060-Vis CHc-_vis CHc M 4 X  16_Défaut_sldprt.STL"  UnitType=Custom  ExtGeomFileUnits=mm  StepReaderType=HEX  ExportConvexHullGeometry=off  InertiaType=Custom  Mass=0.00033190900000000002  MassUnits=kg  CenterOfMass=[0 1.06986e-08 8.0784000000000002]  CenterOfMassUnits=mm  MomentsOfInertia=[0.0127177 0.0127186 0.00128578]  MomentsOfInertiaUnits=kg*mm^2  ProductsOfInertia=[0 0 -6.1878200000000004e-08]  ProductsOfInertiaUnits=kg*mm^2  BasedOnType=Density  Density=1000  DensityUnits=kg/(m^3)  DoExposeReferenceFrame=on  SerializedFrames=<Frames/>  GraphicType=FromGeometry  MarkerShape=Sphere  MarkerSize=10  MarkerSizeUnits=m  GraphicVisPropType=SimpleVisualProperties  GraphicDiffuseColor=[0.792157 0.819608 0.933333]  GraphicSpecularColor=[0.5 0.5 0.5 1.0]  GraphicAmbientColor=[0.15 0.15 0.15 1.0]  GraphicEmissiveColor=[0.0 0.0 0.0 1.0]  GraphicShininess=75  GraphicOpacity=1
  F : PMIOPort  Side=Left
  connections:
  F/RConn1 -- ReferenceFrame/RConn1 -- Solid/RConn1

== system Table_airbus_v1/Modèle mécanique/Table/table_1_RIGID/x15060_M_01002_Ens_cadre_Default_1_RIGID/x15060_M_01004_Ens_barre_de_cadre_1_Default_2_RIGID/x15060_M_01041_Plaquette_sur_glissiere_AA_DEFAULT_1_RIGID ==
  ReferenceFrame : sm_lib/Frames and Transforms/Reference Frame
  Solid : sm_lib/Body Elements/File Solid  ExtGeomFileName=15060-M-01041-Plaquette sur glissiere_AA - DEFAULT_Défaut_sldprt.STL  UnitType=Custom  ExtGeomFileUnits=mm  StepReaderType=HEX  ExportConvexHullGeometry=off  InertiaType=Custom  Mass=0.066996899999999998  MassUnits=kg  CenterOfMass=[-1.5298499999999999 -0.085960300000000003 4.9779900000000001]  CenterOfMassUnits=mm  MomentsOfInertia=[7.6590700000000007 34.768699999999995 41.3262]  MomentsOfInertiaUnits=kg*mm^2  ProductsOfInertia=[-0.0011722600000000001 -0.039111800000000002 -0.014471899999999999]  ProductsOfInertiaUnits=kg*mm^2  BasedOnType=Density  Density=1000  DensityUnits=kg/(m^3)  DoExposeReferenceFrame=on  SerializedFrames=<Frames/>  GraphicType=FromGeometry  MarkerShape=Sphere  MarkerSize=10  MarkerSizeUnits=m  GraphicVisPropType=SimpleVisualProperties  GraphicDiffuseColor=[0.898039 0.917647 0.929412]  GraphicSpecularColor=[0.5 0.5 0.5 1.0]  GraphicAmbientColor=[0.15 0.15 0.15 1.0]  GraphicEmissiveColor=[0.0 0.0 0.0 1.0]  GraphicShininess=75  GraphicOpacity=1
  F : PMIOPort  Side=Left
  connections:
  F/RConn1 -- ReferenceFrame/RConn1 -- Solid/RConn1
